simulink model "replay_attack"  (R2021a)
settings: Solver=VariableStepAuto  StartTime=0.0  StopTime=10.0  RelTol=1e-3
values from neighbouring files (symbols this model uses):
  max_delay = 1    [attack_setUp.m]
  probability = 2^(-4)    (= 0.0625)    [attack_setUp.m]
  seed_probability = 1    [attack_setUp.m]
settings Model: Creator=uidk9388  LastModifiedBy=uidk9388

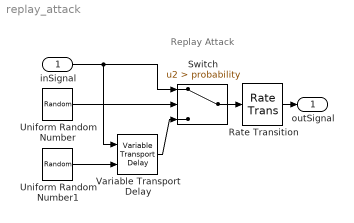
== system replay_attack ==
  note: Replay Attack
  inSignal : Inport
  Rate Transition : RateTransition  OutPortSampleTime=Ts
  Switch : Switch  Criteria=u2 > Threshold  Threshold=probability
  Uniform Random Number : UniformRandomNumber  Minimum=0  Seed=seed_probability  SampleTime=0.1
  Uniform Random Number1 : UniformRandomNumber  Minimum=0  Maximum=max_delay  SampleTime=0.1
  Variable Transport Delay : VariableTransportDelay  VariableDelayType=Variable transport delay  MaximumDelay=max_delay
  outSignal : Outport
  wires:
  Switch/1 -> Rate Transition/1
  Uniform Random Number/1 -> Switch/2
  inSignal/1 -> Variable Transport Delay/1, Switch/1
  Variable Transport Delay/1 -> Switch/3
  Rate Transition/1 -> outSignal/1
  Uniform Random Number1/1 -> Variable Transport Delay/2
